simulink model "State_Machine"  (R2021b)
settings: configuration reference "BMS_Sw_CodeGenConfig" (kept outside this file)
undefined symbols (not defined in the file): contactorTime, currentFactor, CV_Gain, HighTempLimit, I_cc, LowTempLimit, MaxCellVoltThrsld, noCurrent, OverCellVoltageLimit, SnsrFltThld, timeoutContactor, timeoutCurrent, UnderCellVoltageLimit, voltThreshold, vRatio
settings Model: DataDictionary=DD_State_Machine.sldd  EnableAccessToBaseWorkspace=off  ExtModeTrigDuration=5  Creator=Chirag Patel  LastModifiedBy=lordx
settings ConfigSetRef: SourceName=BMS_Sw_CodeGenConfig

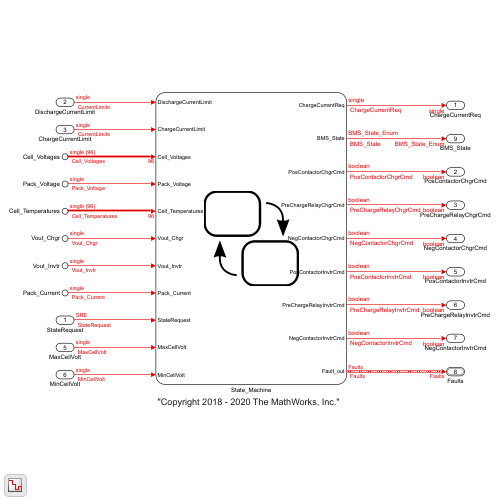
[thumbnail: Simulink's stored preview of the top-level diagram]
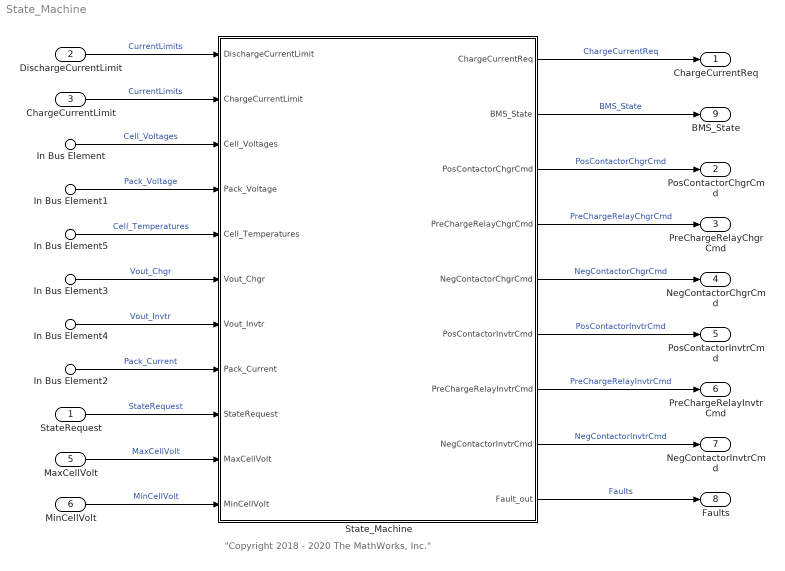
== system State_Machine ==
  note: "Copyright 2018 - 2020 The MathWorks, Inc."
  StateRequest : Inport  OutDataTypeStr=Enum: SRE  PortDimensions=1  SampleTime=[0.10000000000000001,0]
  DischargeCurrentLimit : Inport  Port=2
  ChargeCurrentLimit : Inport  Port=3
  In Bus Element : Inport  Port=4  PortName=BMS_Input  Element=Cell_Voltages
  In Bus Element1 : Inport  Port=4  PortName=BMS_Input  Element=Pack_Voltage
  In Bus Element2 : Inport  Port=4  PortName=BMS_Input  Element=Pack_Current
  In Bus Element3 : Inport  Port=4  PortName=BMS_Input  Element=Vout_Chgr
  In Bus Element4 : Inport  Port=4  PortName=BMS_Input  Element=Vout_Invtr
  In Bus Element5 : Inport  Port=4  PortName=BMS_Input  Element=Cell_Temperatures
  MaxCellVolt : Inport  Port=5  OutMin=0  OutMax=5  OutDataTypeStr=single  PortDimensions=1  SampleTime=[0.10000000000000001,0]
  MinCellVolt : Inport  Port=6  OutMin=0  OutMax=5  OutDataTypeStr=single  PortDimensions=1  SampleTime=[0.10000000000000001,0]
  State_Machine : Stateflow chart  TreatAsAtomicUnit=on  VariantControl=(default)
  ChargeCurrentReq : Outport  OutMin=-100  OutMax=100  OutDataTypeStr=single  PortDimensions=1  SampleTime=[0.10000000000000001,0]  VectorParamsAs1DForOutWhenUnconnected=off
  PosContactorChgrCmd : Outport  Port=2  OutMin=0  OutMax=1  OutDataTypeStr=boolean  PortDimensions=1  SampleTime=[0.10000000000000001,0]  VectorParamsAs1DForOutWhenUnconnected=off
  PreChargeRelayChgrCmd : Outport  Port=3  OutMin=0  OutMax=1  OutDataTypeStr=boolean  PortDimensions=1  SampleTime=[0.10000000000000001,0]  VectorParamsAs1DForOutWhenUnconnected=off
  NegContactorChgrCmd : Outport  Port=4  OutMin=0  OutMax=1  OutDataTypeStr=boolean  PortDimensions=1  SampleTime=[0.10000000000000001,0]  VectorParamsAs1DForOutWhenUnconnected=off
  PosContactorInvtrCmd : Outport  Port=5  OutMin=0  OutMax=1  OutDataTypeStr=boolean  PortDimensions=1  SampleTime=[0.10000000000000001,0]  VectorParamsAs1DForOutWhenUnconnected=off
  PreChargeRelayInvtrCmd : Outport  Port=6  OutMin=0  OutMax=1  OutDataTypeStr=boolean  PortDimensions=1  SampleTime=[0.10000000000000001,0]  VectorParamsAs1DForOutWhenUnconnected=off
  NegContactorInvtrCmd : Outport  Port=7  OutMin=0  OutMax=1  OutDataTypeStr=boolean  PortDimensions=1  SampleTime=[0.10000000000000001,0]  VectorParamsAs1DForOutWhenUnconnected=off
  Faults : Outport  Port=8  OutDataTypeStr=Bus: Faults  VectorParamsAs1DForOutWhenUnconnected=off  BusOutputAsStruct=on
  BMS_State : Outport  Port=9  OutDataTypeStr=Enum: BMS_State_Enum  PortDimensions=1  SampleTime=[0.10000000000000001,0]  VectorParamsAs1DForOutWhenUnconnected=off
  wires:
  State_Machine/2(BMS_State) -> BMS_State/1  "BMS_State"
  State_Machine/1(ChargeCurrentReq) -> ChargeCurrentReq/1  "ChargeCurrentReq"
  State_Machine/3(PosContactorChgrCmd) -> PosContactorChgrCmd/1  "PosContactorChgrCmd"
  State_Machine/4(PreChargeRelayChgrCmd) -> PreChargeRelayChgrCmd/1  "PreChargeRelayChgrCmd"
  State_Machine/5(NegContactorChgrCmd) -> NegContactorChgrCmd/1  "NegContactorChgrCmd"
  State_Machine/6(PosContactorInvtrCmd) -> PosContactorInvtrCmd/1  "PosContactorInvtrCmd"
  State_Machine/7(PreChargeRelayInvtrCmd) -> PreChargeRelayInvtrCmd/1  "PreChargeRelayInvtrCmd"
  State_Machine/8(NegContactorInvtrCmd) -> NegContactorInvtrCmd/1  "NegContactorInvtrCmd"
  State_Machine/9(Fault_out) -> Faults/1  "Faults"
  DischargeCurrentLimit/1 -> State_Machine/1(DischargeCurrentLimit)  "CurrentLimits"
  ChargeCurrentLimit/1 -> State_Machine/2(ChargeCurrentLimit)  "CurrentLimits"
  In Bus Element/1 -> State_Machine/3(Cell_Voltages)  "Cell_Voltages"
  MinCellVolt/1 -> State_Machine/11(MinCellVolt)  "MinCellVolt"
  MaxCellVolt/1 -> State_Machine/10(MaxCellVolt)  "MaxCellVolt"
  StateRequest/1 -> State_Machine/9(StateRequest)  "StateRequest"
  In Bus Element2/1 -> State_Machine/8(Pack_Current)  "Pack_Current"
  In Bus Element4/1 -> State_Machine/7(Vout_Invtr)  "Vout_Invtr"
  In Bus Element3/1 -> State_Machine/6(Vout_Chgr)  "Vout_Chgr"
  In Bus Element5/1 -> State_Machine/5(Cell_Temperatures)  "Cell_Temperatures"
  In Bus Element1/1 -> State_Machine/4(Pack_Voltage)  "Pack_Voltage"

== stateflow chart State_Machine/State_Machine ==
  state FaultMonitoring [parallel]
    settings: executionOrder=2
    state MonitorCurrLim [parallel]
      settings: executionOrder=1
      state NoCurrLimFault
      state OverCurrentFault
        en:
        FaultPresent = true;
        Fault_out.OverCurrent=true;
      (default) -> NoCurrLimFault : {FaultPresent = false;
          | Fault_out.OverCurrent=false;}
      NoCurrLimFault -> OverCurrentFault : [duration(((DischargeCurrentLimit - Pack_Current)<single(0.2) || ...
          | (Pack_Current - ChargeCurrentLimit) < single(0.2)) > timeoutCurrent,sec)]
    state MonitorCellVoltage [parallel]
      settings: executionOrder=2
      state OverVoltageFault
        en:
        FaultPresent = true;
        Fault_out.OverVolt = true;
      state NoCellVoltFault
        en,du:
        SumOfVoltages = sum(Cell_Voltages);
        Delta = abs(Pack_Voltage - SumOfVoltages);
      state SensorFaut
        en:
        FaultPresent = true;
        Fault_out.VoltSensor = true;
      state UnderVoltageFault
        en:
        FaultPresent = true;
        Fault_out.UnderVolt = true;
      (default) -> NoCellVoltFault : {FaultPresent = false;
          | Fault_out.OverVolt = false;
          | Fault_out.UnderVolt = false;
          | Fault_out.VoltSensor = false;
          | }
      NoCellVoltFault -> OverVoltageFault [order 1] : [MaxCellVolt >= ...
          | OverCellVoltageLimit]
      NoCellVoltFault -> SensorFaut [order 3] : [Delta >=...
          |  single(SnsrFltThld)]
      NoCellVoltFault -> UnderVoltageFault [order 2] : [MinCellVolt <=...
          |  UnderCellVoltageLimit]
    state MonitorCellTemp [parallel]
      settings: executionOrder=3
      state HighTemperatureFault
        en:
        FaultPresent = true;
        Fault_out.HighTemp = true;
      state NoCellTempFault
        en,du:
        MaxCellTemp = max(Cell_Temperatures);
        MinCellTemp = min(Cell_Temperatures);
      state LowTemperatureFault
        en:
        FaultPresent = true;
        Fault_out.LowTemp = true;
      (default) -> NoCellTempFault : {FaultPresent = false;
          | Fault_out.HighTemp = false;
          | Fault_out.LowTemp = false;}
      NoCellTempFault -> HighTemperatureFault [order 1] : [MaxCellTemp >= HighTempLimit]
      NoCellTempFault -> LowTemperatureFault [order 2] : [MinCellTemp <= LowTempLimit]
  state MainStateMachine [parallel]
    settings: executionOrder=1
    state Charging
      en:
      BMS_State = BMS_State_Enum.BMS_Charging;
      state Init_Mode
        en:
        ChargeModeReq = Charge_Mode_Enum.Init_Mode;
        ChargeCurrentReq = noCurrent;
      state CC_Mode
        en:
        ChargeModeReq = Charge_Mode_Enum.CC_Mode;
        du:
        ChargeCurrentReq = min(I_cc,ChargeCurrentLimit);
      state CV_Mode
        en:
        ChargeModeReq = Charge_Mode_Enum.CV_Mode;
        du:
        ChargeCurrentReq = ChargeCurrentReq - CV_Gain*(MaxCellVolt - MaxCellVoltThrsld);
        ChargeCurrentReq = min(ChargeCurrentReq, ChargeCurrentLimit);
      (default) -> Init_Mode
      CV_Mode -> Init_Mode : [StateRequest ~= SRE.Charging || ...
          | ChargeCurrentReq <= (I_cc/currentFactor)]
      CC_Mode -> Init_Mode [order 1] : [StateRequest ~= SRE.Charging]
      Init_Mode -> CC_Mode : [StateRequest == SRE.Charging && ...
          | MaxCellVolt < voltThreshold]
      CC_Mode -> CV_Mode [order 2] : [MaxCellVolt>=...
          | MaxCellVoltThrsld]
    state Standby
      en:
      BMS_State = ...
      BMS_State_Enum.BMS_Standby;
    state Driving
      en:
      BMS_State = ...
      BMS_State_Enum.BMS_Driving;
    state Fault
      en,du:
      BMS_State = BMS_State_Enum.BMS_Fault;
    (default) -> Standby
    Standby -> (junction 577) [order 1] : [FaultPresent]
    Standby -> Charging [order 2] : [StateRequest ==SRE.Charging...
        | && ChrgCntctState == Contact.Close]
    (junction 577) -> (junction 580)
    Charging -> Standby [order 3] : [StateRequest ~=SRE.Charging...
        |  && ChrgCntctState == Contact.Init]
    Standby -> Driving [order 3] : [StateRequest == SRE.Driving && ...
        | InvtrCntctState == Contact.Close]
    Driving -> Standby [order 3] : [StateRequest ~= SRE.Driving && ...
        | InvtrCntctState == Contact.Init]
    Driving -> Charging [order 2] : [StateRequest == SRE.Charging && ...
        | ChrgCntctState == Contact.Close]
    Charging -> Driving [order 2] : [StateRequest == SRE.Driving && ...
        | InvtrCntctState == Contact.Close]
    Driving -> Fault [order 1] : [FaultPresent]
    Charging -> Fault [order 1] : [FaultPresent]{ChargeCurrentReq = single(0);}
    (junction 580) -> Fault
  state ChargerContactorState [parallel]
    settings: executionOrder=3
    state OpenChgrContactors
      state ClosePreChrgRly
        PreChargeRelayChgrCmd = true;
      state OpenPosCntct
        PosContactorChgrCmd = false;
      state OpenPreChrgRly
        PreChargeRelayChgrCmd = false;
      state OpenNegCntct
        NegContactorChgrCmd = false;
        ChrgCntctState = Contact.Open;
        PreChrgFault = false;
        Fault_out.Charger = false;
      (default) -> ChargerContactorState.OpenChgrContactors.ClosePreChrgRly : {ChrgCntctState = Contact.Init;}
      ChargerContactorState.OpenChgrContactors.ClosePreChrgRly -> ChargerContactorState.OpenChgrContactors.OpenPosCntct : after(contactorTime,msec) % Check for low current
      ChargerContactorState.OpenChgrContactors.OpenPosCntct -> ChargerContactorState.OpenChgrContactors.OpenPreChrgRly : after(contactorTime,msec)
      ChargerContactorState.OpenChgrContactors.OpenPreChrgRly -> ChargerContactorState.OpenChgrContactors.OpenNegCntct : after(contactorTime,msec)
    state CloseChgrContactors
      state CloseNegCntct
        NegContactorChgrCmd = true;
      state ClosePreChrgRly
        PreChargeRelayChgrCmd = true;
      state ClosePosCntct
        PosContactorChgrCmd = true;
      state OpenPreChrgRly
        PreChargeRelayChgrCmd = false;
        ChrgCntctState = Contact.Close;
      state PreChrgFlt
        PreChrgFault = true;
        Fault_out.Charger = true;
      (default) -> ChargerContactorState.CloseChgrContactors.CloseNegCntct : {ChrgCntctState = Contact.Init;}
      ChargerContactorState.CloseChgrContactors.CloseNegCntct -> ChargerContactorState.CloseChgrContactors.ClosePreChrgRly : after(contactorTime,msec)
      ChargerContactorState.CloseChgrContactors.ClosePreChrgRly -> (junction 564) [order 2]
      (junction 564) -> (junction 566) : after(timeoutContactor,sec)
          | % Check timeout
      ChargerContactorState.CloseChgrContactors.ClosePreChrgRly -> ChargerContactorState.CloseChgrContactors.ClosePosCntct [order 1] : [Vout_Chgr/Pack_Voltage >=vRatio]
      ChargerContactorState.CloseChgrContactors.ClosePosCntct -> ChargerContactorState.CloseChgrContactors.OpenPreChrgRly : after(contactorTime,msec)
      (junction 566) -> ChargerContactorState.CloseChgrContactors.PreChrgFlt
    (default) -> OpenChgrContactors : {ChrgCntctState = Contact.Init;
        | PreChrgFault = false;
        | Fault_out.Charger = false;}
    CloseChgrContactors -> OpenChgrContactors : [StateRequest ~= SRE.Charging || ...
        | FaultPresent]
    OpenChgrContactors -> CloseChgrContactors : [StateRequest == SRE.Charging && ...
        | InvtrCntctState == Contact.Open && ...
        | ~FaultPresent]
  state InverterContactorState [parallel]
    settings: executionOrder=4
    state CloseInvtrContactors
      state CloseNegCntct
        NegContactorInvtrCmd = true;
      state ClosePreChrgRly
        PreChargeRelayInvtrCmd = true;
      state ClosePosCntct
        PosContactorInvtrCmd = true;
      state OpenPreChrgRly
        PreChargeRelayInvtrCmd = false;
        InvtrCntctState = Contact.Close;
      state PreChrgFlt
        PreChrgFault = true;
        Fault_out.Inverter = true;
      (default) -> InverterContactorState.CloseInvtrContactors.CloseNegCntct : {InvtrCntctState = Contact.Init;}
      InverterContactorState.CloseInvtrContactors.CloseNegCntct -> InverterContactorState.CloseInvtrContactors.ClosePreChrgRly : after(contactorTime,msec)
      InverterContactorState.CloseInvtrContactors.ClosePreChrgRly -> (junction 569) [order 2]
      (junction 569) -> (junction 570) : after(timeoutContactor,sec)
          | % Check timeout
      InverterContactorState.CloseInvtrContactors.ClosePreChrgRly -> InverterContactorState.CloseInvtrContactors.ClosePosCntct [order 1] : [Vout_Invtr/Pack_Voltage >=vRatio]
      InverterContactorState.CloseInvtrContactors.ClosePosCntct -> InverterContactorState.CloseInvtrContactors.OpenPreChrgRly : after(contactorTime,msec)
      (junction 570) -> InverterContactorState.CloseInvtrContactors.PreChrgFlt
    state OpenInvtrContactors
      state ClosePreChrgRly
        PreChargeRelayInvtrCmd = true;
      state OpenPosCntct
        PosContactorInvtrCmd = false;
      state OpenPreChrgRly
        PreChargeRelayInvtrCmd = false;
      state OpenNegCntct
        NegContactorInvtrCmd = false;
        InvtrCntctState = Contact.Open;
        PreChrgFault = false;
        Fault_out.Inverter = false;
      (default) -> InverterContactorState.OpenInvtrContactors.ClosePreChrgRly : {InvtrCntctState = Contact.Init;}
      InverterContactorState.OpenInvtrContactors.ClosePreChrgRly -> InverterContactorState.OpenInvtrContactors.OpenPosCntct : after(contactorTime,msec) % Check for low current
      InverterContactorState.OpenInvtrContactors.OpenPosCntct -> InverterContactorState.OpenInvtrContactors.OpenPreChrgRly : after(contactorTime,msec)
      InverterContactorState.OpenInvtrContactors.OpenPreChrgRly -> InverterContactorState.OpenInvtrContactors.OpenNegCntct : after(contactorTime,msec)
    (default) -> OpenInvtrContactors : {InvtrCntctState =Contact.Init;
        | PreChrgFault = false;
        | Fault_out.Inverter = false;}
    CloseInvtrContactors -> OpenInvtrContactors : [StateRequest ~= SRE.Driving || ...
        | FaultPresent]
    OpenInvtrContactors -> CloseInvtrContactors : [StateRequest == SRE.Driving && ...
        | ChrgCntctState == Contact.Open && ...
        | ~FaultPresent]
  data: DischargeCurrentLimit input single; ChargeCurrentLimit input; Cell_Voltages input single; Pack_Voltage input single; Cell_Temperatures input single; Vout_Chgr input single; Vout_Invtr input single; Pack_Current input single; StateRequest input Enum: SRE; ChargeCurrentReq output; I_cc parameter; MaxCellVolt input single; BMS_State output Enum: BMS_State_Enum =BMS_State_Enum.BMS_Standby; PosContactorChgrCmd output boolean; PreChargeRelayChgrCmd output; NegContactorChgrCmd output; PosContactorInvtrCmd output; PreChargeRelayInvtrCmd output; NegContactorInvtrCmd output; ChrgCntctState local Enum: Contact; InvtrCntctState local Enum: Contact; PreChrgFault local; MaxCellVoltThrsld parameter; FaultPresent local; MinCellVolt input single; MaxCellTemp local; OverCellVoltageLimit parameter; UnderCellVoltageLimit parameter; MinCellTemp local; Delta local; HighTempLimit parameter; LowTempLimit parameter; SnsrFltThld parameter; SumOfVoltages local; CV_Gain parameter; ChargeModeReq local Enum: Charge_Mode_Enum =Charge_Mode_Enum.Init_Mode; MonitorCurrLimMode local Enum: MonitorCurrLimModeType; MonitorCellVoltageMode local Enum: MonitorCellVoltageModeType; MonitorCellTempMode local Enum: MonitorCellTempModeType; Fault_out output Bus: Faults; contactorTime parameter uint16; timeoutContactor parameter uint8; timeoutCurrent parameter uint8; vRatio parameter single; voltThreshold parameter single; currentFactor parameter single; noCurrent parameter single
